simulink model "NOP"  (R2017a)
settings: Solver=VariableStepAuto  StartTime=0.0  StopTime=inf  RelTol=1e-3
values from neighbouring files (symbols this model uses):
  N = sqrt(1-M*M)    [untitled.m]
libraries: mblibv1 x18, simulink x4
settings Model: Creator=Admin  LastModifiedBy=Admin
settings SimMechanicsCC: VisOnUpdateDiagram=on  VisDuringSimulation=on

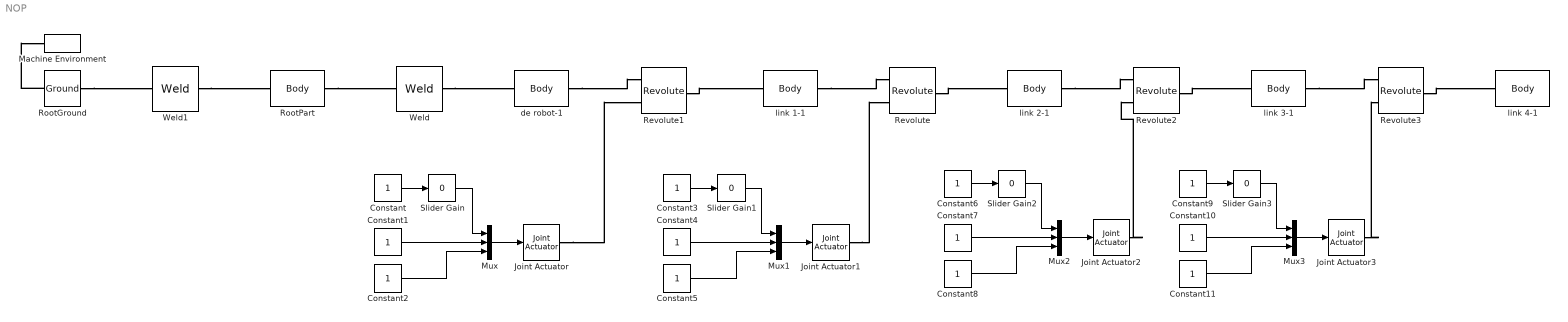
== system NOP ==
  Constant{,1..11} (12 alike) : Constant
  Joint Actuator{,1..3} (4 alike) : mblibv1/Sensors &  Actuators/Joint Actuator  UpdateFromCAD=off  PhysicalDomain=Mechanical  PortType=blob  ActuationStyle=Motion  AngleUnits=deg  ArcVelocityUnits=deg/s  ArcAccelerationUnits=deg/s^2  CoordPositionUnits=m  VelocityUnits=m/s  AccelerationUnits=m/s^2  ForceUnits=N  TorqueUnits=N*m  ActiveIO=on  Width=3  DialogClass=MechanicalActuatorBlock  Primitive=R1  ReferenceFrame=Absolute (World)
      settings: SourceProductName=Simscape Multibody  SourceProductBaseCode=MS
  Machine Environment : mblibv1/Bodies/Machine Environment  PortType=env  PhysicalDomain=Mechanical  DialogTemplateClass=MECH.MachineEnvironment  SyncWhenCopied=off  Gravity=[0 -9.81 0]  GravityUnits=m/s^2  GravityAsSignal=off  Dimensionality=Auto-detect  AnalysisType=Forward dynamics  LinearAssemblyTolerance=1e-3  LinearAssemblyToleranceUnits=m  AngularAssemblyTolerance=1e-3  AngularAssemblyToleranceUnits=rad  ConstraintSolverType=Stabilizing  ConstraintRelTolerance=1e-4  ConstraintAbsTolerance=1e-4  UseRobustSingularityHandling=off  RedundancyAnalysisToleranceType=Automatically select tolerance  RedundancyAnalysisTolerance=1e-14  StatePerturbationType=Fixed  PerturbationSize=1e-5  VisualizeMachine=on  BodyVisualizationType=Use model default body geometries  BodyColorSelMode=Use model default  DefaultBodyColor=[1 0 0]
      settings: SourceProductName=Simscape Multibody  SourceProductBaseCode=MS
  Mux{,1..3} (4 alike) : Mux  Inputs=3
  Revolute : mblibv1/Joints/Revolute  LConnTagsString=__newl0|SA1  RConnTagsString=__newr0  UpdateFromCAD=on  PMImportedID=link 1-1:-:link 2-1  NumSAPorts=1  CutJoint=off  MarkAsCut=off  Primitives=prismatic  PrimitiveProps=R1$World$[-0.000159407,-1,0]$revolute  DialogClass=JointBlock  R1Axis=[-0.000159407,-1,0]
      settings: SourceProductName=Simscape Multibody  SourceProductBaseCode=MS
  Revolute1 : mblibv1/Joints/Revolute  LConnTagsString=__newl0|SA1  RConnTagsString=__newr0  UpdateFromCAD=on  PMImportedID=de robot-1:-:link 1-1  NumSAPorts=1  CutJoint=off  MarkAsCut=off  Primitives=prismatic  PrimitiveProps=R1$World$[0,0,-1]$revolute  DialogClass=JointBlock  R1Axis=[0,0,-1]
      settings: SourceProductName=Simscape Multibody  SourceProductBaseCode=MS
  Revolute2 : mblibv1/Joints/Revolute  LConnTagsString=__newl0|SA1  RConnTagsString=__newr0  UpdateFromCAD=on  PMImportedID=link 2-1:-:link 3-1  NumSAPorts=1  CutJoint=off  MarkAsCut=off  Primitives=prismatic  PrimitiveProps=R1$World$[-0.000159407,-1,0]$revolute  DialogClass=JointBlock  R1Axis=[-0.000159407,-1,0]
      settings: SourceProductName=Simscape Multibody  SourceProductBaseCode=MS
  Revolute3 : mblibv1/Joints/Revolute  LConnTagsString=__newl0|SA1  RConnTagsString=__newr0  UpdateFromCAD=on  PMImportedID=link 3-1:-:link 4-1  NumSAPorts=1  CutJoint=off  MarkAsCut=off  Primitives=prismatic  PrimitiveProps=R1$World$[-0.000159407,-1,0]$revolute  DialogClass=JointBlock  R1Axis=[-0.000159407,-1,0]
      settings: SourceProductName=Simscape Multibody  SourceProductBaseCode=MS
  RootGround : mblibv1/Bodies/Ground  UpdateFromCAD=on  PMImportedID=RootGround  LeftPortType=env  RightPortType=workingframe  PhysicalDomain=Mechanical  DialogClass=GroundBlock  CoordPosition=[0.0111258,-0.0001479,0.0686258]  CoordPositionUnits=m  StateVectorMgrId=0  MachineId=[1 0]  ShowEnvPort=on  ParameterChecksum=[207017882, 1327668099, 3122716516, 2405378770]  TopologyChecksum=[3601677968, 9615495, 3079123065, 1389597935]
      settings: SourceProductName=Simscape Multibody  SourceProductBaseCode=MS
  RootPart : mblibv1/Bodies/Body  LConnTagsString=CS3  RConnTagsString=CS2  UpdateFromCAD=on  PMImportedID=NOP/RootPart  DialogClass=MechanicalBodyBlock  Mass=0  MassUnits=kg  InertiaUnits=kg*m^2  Inertia=[0,0,0;0,0,0;0,0,0]  Shape=Cylinder  ShapeDims=[1 1]  ShapeUnits=m  ShapeUse=false  Density=1  DensityUnits=kg/m^3  DensityUse=false  GraphicsMode=MACHINE_DEFAULT  BodyColorSelMode=MACHINE_DEFAULT  BodyColor=[1;0;0]  AttachedToCS=CS1  CG=Right$CG$[0.0111258 -0.0001479 0.0686258]$WORLD$WORLD$m$[1 0 0;0 1 0;0 0 1]$3x3 Transform$rad$WORLD$false$NOP/RootPart::CG(AUTOGEN)  WorkingFrames=Right$CS1$[0 0 0]$WORLD$WORLD$m$[1 0 0;0 1 0;0 0 1]$3x3 Transform$rad$WORLD$false$NOP/RootPart::CS1(AUTOGEN)#Right$CS2$[0.0226523 -0.000305703 0.0198925]$WORLD$WORLD$m$[1 0 0;0 1 0;0 0 1]$3x3 Transform$rad$WORLD$true$NOP/RootPart:-:de robot-1::NOP/RootPart(AUTOGEN)#Left$CS3$[0.0111258 -0.0001479 0.0686258]$WORLD$WORLD$m$[1 0 0;0 1 0;0 0 1]$3x3 Transform$rad$WORLD$true$NOP/RootPart:-:RootGround::NOP/RootPart(AUTOGEN)  CGPos=[0.0111258 -0.0001479 0.0686258]  CGRot=[1 0 0;0 1 0;0 0 1]  CS0Pos=[]  CS0Rot=[]  CS1Pos=[0 0 0]  CS1Rot=[1 0 0;0 1 0;0 0 1]  CS2Pos=[0.0226523 -0.000305703 0.0198925]  CS2Rot=[1 0 0;0 1 0;0 0 1]  CS3Pos=[0.0111258 -0.0001479 0.0686258]  CS3Rot=[1 0 0;0 1 0;0 0 1]  CS4Pos=[]  CS4Rot=[]  CS5Pos=[]  CS5Rot=[]  CS6Pos=[]  CS6Rot=[]  CS7Pos=[]  CS7Rot=[]  CS8Pos=[]  CS8Rot=[]  CS9Pos=[]  CS9Rot=[]  CS10Pos=[]  CS10Rot=[]  CS11Pos=[]  CS11Rot=[]  CS12Pos=[]  CS12Rot=[]  CS13Pos=[]  CS13Rot=[]  CS14Pos=[]  CS14Rot=[]  CS15Pos=[]  CS15Rot=[]  CS16Pos=[]  CS16Rot=[]  CS17Pos=[]  CS17Rot=[]  CS18Pos=[]  CS18Rot=[]  CS19Pos=[]  CS19Rot=[]  CS20Pos=[]  CS20Rot=[]
      settings: SourceProductName=Simscape Multibody  SourceProductBaseCode=MS
  Slider Gain{,1..3} (4 alike) : simulink/Math Operations/Slider Gain  gain=0  low=-180  high=180
  Weld : mblibv1/Joints/Weld  LConnTagsString=__newl0  RConnTagsString=__newr0  UpdateFromCAD=on  PMImportedID=NOP/RootPart:-:de robot-1  NumSAPorts=0  CutJoint=off  MarkAsCut=off  Primitives=weld  PrimitiveProps=W$WORLD$[0.57735,0.57735,0.57735]$weld  DialogClass=JointBlock  WAxis=[0.57735,0.57735,0.57735]
      settings: SourceProductName=Simscape Multibody  SourceProductBaseCode=MS
  Weld1 : mblibv1/Joints/Weld  LConnTagsString=__newl0  RConnTagsString=__newr0  UpdateFromCAD=on  PMImportedID=NOP/RootPart:-:RootGround  NumSAPorts=0  CutJoint=off  MarkAsCut=off  Primitives=weld  PrimitiveProps=W$WORLD$[0.57735,0.57735,0.57735]$weld  DialogClass=JointBlock  WAxis=[0.57735,0.57735,0.57735]
      settings: SourceProductName=Simscape Multibody  SourceProductBaseCode=MS
  de robot-1 : mblibv1/Bodies/Body  LConnTagsString=CS2  RConnTagsString=CS3  UpdateFromCAD=on  PMImportedID=de robot-1  DialogClass=MechanicalBodyBlock  Mass=0.451279  MassUnits=kg  InertiaUnits=kg*m^2  Inertia=[0.000359034,1.00878e-05,4.29188e-05;1.00878e-05,0.000788173,6.73597e-07;4.29188e-05,6.73597e-07,0.000996356]  Shape=Cylinder  ShapeDims=[1 1]  ShapeUnits=m  ShapeUse=false  Density=1  DensityUnits=kg/m^3  DensityUse=false  GraphicsMode=GFXFILE  GraphicsFileName=NOP - de robot-1.STL  BodyColorSelMode=COLORPALETTE  BodyColor=[0.909804;0.443137;0.0313725]  AttachedToCS=CS1  CG=Right$CG$[0.0226523 -0.000305703 0.0198925]$WORLD$WORLD$m$[1 0 0;0 1 0;0 0 1]$3x3 Transform$rad$WORLD$false$de robot-1::CG(AUTOGEN)  WorkingFrames=Right$CS1$[0 0 0]$WORLD$WORLD$m$[1 0 0;0 1 0;0 0 1]$3x3 Transform$rad$WORLD$false$de robot-1::CS1(AUTOGEN)#Left$CS2$[0.0226523 -0.000305703 0.0198925]$WORLD$WORLD$m$[1 0 0;0 1 0;0 0 1]$3x3 Transform$rad$WORLD$true$NOP/RootPart:-:de robot-1::de robot-1(AUTOGEN)#Right$CS3$[0 0 0.055]$WORLD$WORLD$m$[1 0 0;0 1 0;0 0 1]$3x3 Transform$rad$WORLD$true$de robot-1:-:link 1-1::de robot-1(AUTOGEN)  CGPos=[0.0226523 -0.000305703 0.0198925]  CGRot=[1 0 0;0 1 0;0 0 1]  CS0Pos=[]  CS0Rot=[]  CS1Pos=[0 0 0]  CS1Rot=[1 0 0;0 1 0;0 0 1]  CS2Pos=[0.0226523 -0.000305703 0.0198925]  CS2Rot=[1 0 0;0 1 0;0 0 1]  CS3Pos=[0 0 0.055]  CS3Rot=[1 0 0;0 1 0;0 0 1]  CS4Pos=[]  CS4Rot=[]  CS5Pos=[]  CS5Rot=[]  CS6Pos=[]  CS6Rot=[]  CS7Pos=[]  CS7Rot=[]  CS8Pos=[]  CS8Rot=[]  CS9Pos=[]  CS9Rot=[]  CS10Pos=[]  CS10Rot=[]  CS11Pos=[]  CS11Rot=[]  CS12Pos=[]  CS12Rot=[]  CS13Pos=[]  CS13Rot=[]  CS14Pos=[]  CS14Rot=[]  CS15Pos=[]  CS15Rot=[]  CS16Pos=[]  CS16Rot=[]  CS17Pos=[]  CS17Rot=[]  CS18Pos=[]  CS18Rot=[]  CS19Pos=[]  CS19Rot=[]  CS20Pos=[]  CS20Rot=[]
      settings: SourceProductName=Simscape Multibody  SourceProductBaseCode=MS
  link 1-1 : mblibv1/Bodies/Body  LConnTagsString=CS3  RConnTagsString=CS2  UpdateFromCAD=on  PMImportedID=link 1-1  DialogClass=MechanicalBodyBlock  Mass=0.299899  MassUnits=kg  InertiaUnits=kg*m^2  Inertia=[0.00046491,-0.00019294,-6.39146e-10;-0.00019294,0.000282392,-1.43061e-09;-6.39146e-10,-1.43061e-09,0.000584388]  Shape=Cylinder  ShapeDims=[1 1]  ShapeUnits=m  ShapeUse=false  Density=1  DensityUnits=kg/m^3  DensityUse=false  GraphicsMode=GFXFILE  GraphicsFileName=NOP - link 1-1.STL  BodyColorSelMode=COLORPALETTE  BodyColor=[1;1;0.501961]  AttachedToCS=CS1  CG=Right$CG$[-0.0198194 3.72349e-06 0.0955822]$WORLD$WORLD$m$[1 0 0.000159407;-0.000159407 0 1;0 -1 0]$3x3 Transform$rad$WORLD$false$link 1-1::CG(AUTOGEN)  WorkingFrames=Right$CS1$[-0.05 7.97034e-06 0.145]$WORLD$WORLD$m$[1 0 0.000159407;-0.000159407 0 1;0 -1 0]$3x3 Transform$rad$WORLD$false$link 1-1::CS1(AUTOGEN)#Right$CS2$[-0.0500018 -0.011492 0.145]$WORLD$WORLD$m$[1 0 0;0 1 0;0 0 1]$3x3 Transform$rad$WORLD$true$link 1-1:-:link 2-1::link 1-1(AUTOGEN)#Left$CS3$[0 0 0.055]$WORLD$WORLD$m$[1 0 0;0 1 0;0 0 1]$3x3 Transform$rad$WORLD$true$de robot-1:-:link 1-1::link 1-1(AUTOGEN)  CGPos=[-0.0198194 3.72349e-06 0.0955822]  CGRot=[1 0 0.000159407;-0.000159407 0 1;0 -1 0]  CS0Pos=[]  CS0Rot=[]  CS1Pos=[-0.05 7.97034e-06 0.145]  CS1Rot=[1 0 0.000159407;-0.000159407 0 1;0 -1 0]  CS2Pos=[-0.0500018 -0.011492 0.145]  CS2Rot=[1 0 0;0 1 0;0 0 1]  CS3Pos=[0 0 0.055]  CS3Rot=[1 0 0;0 1 0;0 0 1]  CS4Pos=[]  CS4Rot=[]  CS5Pos=[]  CS5Rot=[]  CS6Pos=[]  CS6Rot=[]  CS7Pos=[]  CS7Rot=[]  CS8Pos=[]  CS8Rot=[]  CS9Pos=[]  CS9Rot=[]  CS10Pos=[]  CS10Rot=[]  CS11Pos=[]  CS11Rot=[]  CS12Pos=[]  CS12Rot=[]  CS13Pos=[]  CS13Rot=[]  CS14Pos=[]  CS14Rot=[]  CS15Pos=[]  CS15Rot=[]  CS16Pos=[]  CS16Rot=[]  CS17Pos=[]  CS17Rot=[]  CS18Pos=[]  CS18Rot=[]  CS19Pos=[]  CS19Rot=[]  CS20Pos=[]  CS20Rot=[]
      settings: SourceProductName=Simscape Multibody  SourceProductBaseCode=MS
  link 2-1 : mblibv1/Bodies/Body  LConnTagsString=CS2  RConnTagsString=CS3  UpdateFromCAD=on  PMImportedID=link 2-1  DialogClass=MechanicalBodyBlock  Mass=0.110064  MassUnits=kg  InertiaUnits=kg*m^2  Inertia=[2.18833e-05,-1.87351e-06,-1.05679e-12;-1.87351e-06,0.000106749,1.58957e-11;-1.05679e-12,1.58957e-11,0.000107667]  Shape=Cylinder  ShapeDims=[1 1]  ShapeUnits=m  ShapeUse=false  Density=1  DensityUnits=kg/m^3  DensityUse=false  GraphicsMode=GFXFILE  GraphicsFileName=NOP - link 2-1.STL  BodyColorSelMode=COLORPALETTE  BodyColor=[1;0.501961;0.501961]  AttachedToCS=CS1  CG=Right$CG$[-0.00936915 1.49367e-06 0.146009]$WORLD$WORLD$m$[0.998901 0.0468759 0.000159407;-0.000159231 -7.47233e-06 1;0.0468759 -0.998901 0]$3x3 Transform$rad$WORLD$false$link 2-1::CG(AUTOGEN)  WorkingFrames=Right$CS1$[0.0399723 -6.37184e-06 0.147235]$WORLD$WORLD$m$[0.998901 0.0468759 0.000159407;-0.000159231 -7.47233e-06 1;0.0468759 -0.998901 0]$3x3 Transform$rad$WORLD$false$link 2-1::CS1(AUTOGEN)#Left$CS2$[-0.0500018 -0.011492 0.145]$WORLD$WORLD$m$[1 0 0;0 1 0;0 0 1]$3x3 Transform$rad$WORLD$true$link 1-1:-:link 2-1::link 2-1(AUTOGEN)#Right$CS3$[0.0399768 0.0284936 0.147235]$WORLD$WORLD$m$[1 0 0;0 1 0;0 0 1]$3x3 Transform$rad$WORLD$true$link 2-1:-:link 3-1::link 2-1(AUTOGEN)  CGPos=[-0.00936915 1.49367e-06 0.146009]  CGRot=[0.998901 0.0468759 0.000159407;-0.000159231 -7.47233e-06 1;0.0468759 -0.998901 0]  CS0Pos=[]  CS0Rot=[]  CS1Pos=[0.0399723 -6.37184e-06 0.147235]  CS1Rot=[0.998901 0.0468759 0.000159407;-0.000159231 -7.47233e-06 1;0.0468759 -0.998901 0]  CS2Pos=[-0.0500018 -0.011492 0.145]  CS2Rot=[1 0 0;0 1 0;0 0 1]  CS3Pos=[0.0399768 0.0284936 0.147235]  CS3Rot=[1 0 0;0 1 0;0 0 1]  CS4Pos=[]  CS4Rot=[]  CS5Pos=[]  CS5Rot=[]  CS6Pos=[]  CS6Rot=[]  CS7Pos=[]  CS7Rot=[]  CS8Pos=[]  CS8Rot=[]  CS9Pos=[]  CS9Rot=[]  CS10Pos=[]  CS10Rot=[]  CS11Pos=[]  CS11Rot=[]  CS12Pos=[]  CS12Rot=[]  CS13Pos=[]  CS13Rot=[]  CS14Pos=[]  CS14Rot=[]  CS15Pos=[]  CS15Rot=[]  CS16Pos=[]  CS16Rot=[]  CS17Pos=[]  CS17Rot=[]  CS18Pos=[]  CS18Rot=[]  CS19Pos=[]  CS19Rot=[]  CS20Pos=[]  CS20Rot=[]
      settings: SourceProductName=Simscape Multibody  SourceProductBaseCode=MS
  link 3-1 : mblibv1/Bodies/Body  LConnTagsString=CS2  RConnTagsString=CS3  UpdateFromCAD=on  PMImportedID=link 3-1  DialogClass=MechanicalBodyBlock  Mass=0.0552352  MassUnits=kg  InertiaUnits=kg*m^2  Inertia=[7.24142e-06,-1.609e-13,6.63424e-14;-1.609e-13,6.73724e-05,6.26587e-11;6.63424e-14,6.26587e-11,6.37429e-05]  Shape=Cylinder  ShapeDims=[1 1]  ShapeUnits=m  ShapeUse=false  Density=1  DensityUnits=kg/m^3  DensityUse=false  GraphicsMode=GFXFILE  GraphicsFileName=NOP - link 3-1.STL  BodyColorSelMode=COLORPALETTE  BodyColor=[0.501961;1;0.501961]  AttachedToCS=CS1  CG=Right$CG$[0.0895722 -1.42784e-05 0.147782]$WORLD$WORLD$m$[0.999939 0.0110341 0.000159407;-0.000159397 -1.75891e-06 1;0.0110341 -0.999939 0]$3x3 Transform$rad$WORLD$false$link 3-1::CG(AUTOGEN)  WorkingFrames=Right$CS1$[0.147966 -2.35867e-05 0.148426]$WORLD$WORLD$m$[0.999939 0.0110341 0.000159407;-0.000159397 -1.75891e-06 1;0.0110341 -0.999939 0]$3x3 Transform$rad$WORLD$false$link 3-1::CS1(AUTOGEN)#Left$CS2$[0.0399768 0.0284936 0.147235]$WORLD$WORLD$m$[1 0 0;0 1 0;0 0 1]$3x3 Transform$rad$WORLD$true$link 2-1:-:link 3-1::link 3-1(AUTOGEN)#Right$CS3$[0.147965 -0.00602359 0.148426]$WORLD$WORLD$m$[1 0 0;0 1 0;0 0 1]$3x3 Transform$rad$WORLD$true$link 3-1:-:link 4-1::link 3-1(AUTOGEN)  CGPos=[0.0895722 -1.42784e-05 0.147782]  CGRot=[0.999939 0.0110341 0.000159407;-0.000159397 -1.75891e-06 1;0.0110341 -0.999939 0]  CS0Pos=[]  CS0Rot=[]  CS1Pos=[0.147966 -2.35867e-05 0.148426]  CS1Rot=[0.999939 0.0110341 0.000159407;-0.000159397 -1.75891e-06 1;0.0110341 -0.999939 0]  CS2Pos=[0.0399768 0.0284936 0.147235]  CS2Rot=[1 0 0;0 1 0;0 0 1]  CS3Pos=[0.147965 -0.00602359 0.148426]  CS3Rot=[1 0 0;0 1 0;0 0 1]  CS4Pos=[]  CS4Rot=[]  CS5Pos=[]  CS5Rot=[]  CS6Pos=[]  CS6Rot=[]  CS7Pos=[]  CS7Rot=[]  CS8Pos=[]  CS8Rot=[]  CS9Pos=[]  CS9Rot=[]  CS10Pos=[]  CS10Rot=[]  CS11Pos=[]  CS11Rot=[]  CS12Pos=[]  CS12Rot=[]  CS13Pos=[]  CS13Rot=[]  CS14Pos=[]  CS14Rot=[]  CS15Pos=[]  CS15Rot=[]  CS16Pos=[]  CS16Rot=[]  CS17Pos=[]  CS17Rot=[]  CS18Pos=[]  CS18Rot=[]  CS19Pos=[]  CS19Rot=[]  CS20Pos=[]  CS20Rot=[]
      settings: SourceProductName=Simscape Multibody  SourceProductBaseCode=MS
  link 4-1 : mblibv1/Bodies/Body  LConnTagsString=CS2  UpdateFromCAD=on  PMImportedID=link 4-1  DialogClass=MechanicalBodyBlock  Mass=0.0126078  MassUnits=kg  InertiaUnits=kg*m^2  Inertia=[6.55181e-07,0,0;0,2.19709e-06,0;0,0,2.19932e-06]  Shape=Cylinder  ShapeDims=[1 1]  ShapeUnits=m  ShapeUse=false  Density=1  DensityUnits=kg/m^3  DensityUse=false  GraphicsMode=GFXFILE  GraphicsFileName=NOP - link 4-1.STL  BodyColorSelMode=COLORPALETTE  BodyColor=[1;1;0.752941]  AttachedToCS=CS1  CG=Right$CG$[0.169879 4.2096e-06 0.149429]$WORLD$WORLD$m$[0.998954 0.0457256 0.000159407;-0.00015924 -7.28896e-06 1;0.0457256 -0.998954 0]$3x3 Transform$rad$WORLD$false$link 4-1::CG(AUTOGEN)  WorkingFrames=Right$CS1$[0.2104 -2.24983e-06 0.151284]$WORLD$WORLD$m$[0.998954 0.0457256 0.000159407;-0.00015924 -7.28896e-06 1;0.0457256 -0.998954 0]$3x3 Transform$rad$WORLD$false$link 4-1::CS1(AUTOGEN)#Left$CS2$[0.147965 -0.00602359 0.148426]$WORLD$WORLD$m$[1 0 0;0 1 0;0 0 1]$3x3 Transform$rad$WORLD$true$link 3-1:-:link 4-1::link 4-1(AUTOGEN)  CGPos=[0.169879 4.2096e-06 0.149429]  CGRot=[0.998954 0.0457256 0.000159407;-0.00015924 -7.28896e-06 1;0.0457256 -0.998954 0]  CS0Pos=[]  CS0Rot=[]  CS1Pos=[0.2104 -2.24983e-06 0.151284]  CS1Rot=[0.998954 0.0457256 0.000159407;-0.00015924 -7.28896e-06 1;0.0457256 -0.998954 0]  CS2Pos=[0.147965 -0.00602359 0.148426]  CS2Rot=[1 0 0;0 1 0;0 0 1]  CS3Pos=[]  CS3Rot=[]  CS4Pos=[]  CS4Rot=[]  CS5Pos=[]  CS5Rot=[]  CS6Pos=[]  CS6Rot=[]  CS7Pos=[]  CS7Rot=[]  CS8Pos=[]  CS8Rot=[]  CS9Pos=[]  CS9Rot=[]  CS10Pos=[]  CS10Rot=[]  CS11Pos=[]  CS11Rot=[]  CS12Pos=[]  CS12Rot=[]  CS13Pos=[]  CS13Rot=[]  CS14Pos=[]  CS14Rot=[]  CS15Pos=[]  CS15Rot=[]  CS16Pos=[]  CS16Rot=[]  CS17Pos=[]  CS17Rot=[]  CS18Pos=[]  CS18Rot=[]  CS19Pos=[]  CS19Rot=[]  CS20Pos=[]  CS20Rot=[]
      settings: SourceProductName=Simscape Multibody  SourceProductBaseCode=MS
  wires:
  Slider Gain/1 -> Mux/1
  Mux/1 -> Joint Actuator/1
  Constant1/1 -> Mux/2
  Constant2/1 -> Mux/3
  Constant/1 -> Slider Gain/1
  Slider Gain1/1 -> Mux1/1
  Mux1/1 -> Joint Actuator1/1
  Constant4/1 -> Mux1/2
  Constant5/1 -> Mux1/3
  Constant3/1 -> Slider Gain1/1
  Slider Gain2/1 -> Mux2/1
  Mux2/1 -> Joint Actuator2/1
  Constant7/1 -> Mux2/2
  Constant8/1 -> Mux2/3
  Constant6/1 -> Slider Gain2/1
  Slider Gain3/1 -> Mux3/1
  Mux3/1 -> Joint Actuator3/1
  Constant10/1 -> Mux3/2
  Constant11/1 -> Mux3/3
  Constant9/1 -> Slider Gain3/1
  connections:
  RootPart/RConn1 -- Weld/LConn1
  Weld/RConn1 -- de robot-1/LConn1
  link 1-1/RConn1 -- Revolute/LConn1
  Revolute/RConn1 -- link 2-1/LConn1
  de robot-1/RConn1 -- Revolute1/LConn1
  Revolute1/RConn1 -- link 1-1/LConn1
  link 2-1/RConn1 -- Revolute2/LConn1
  Revolute2/RConn1 -- link 3-1/LConn1
  link 3-1/RConn1 -- Revolute3/LConn1
  Revolute3/RConn1 -- link 4-1/LConn1
  RootGround/RConn1 -- Weld1/LConn1
  Weld1/RConn1 -- RootPart/LConn1
  RootGround/LConn1 -- Machine Environment/RConn1
  Joint Actuator/RConn1 -- Revolute1/LConn2
  Joint Actuator1/RConn1 -- Revolute/LConn2
  Joint Actuator2/RConn1 -- Revolute2/LConn2
  Joint Actuator3/RConn1 -- Revolute3/LConn2
